simulink model "Car"  (R2024b)
settings: Solver=ode15s  StartTime=0.0  StopTime=PROFILE_LENGTH  MaxStep=300  RelTol=1e-7
values from neighbouring files (symbols this model uses):
  ACCEL_TOLERANCE = 1    [Setup.m]
  AIR_DENSITY = 1.2    [Setup.m]
  C_ROLLING_RESISTANCE = .0025    (= 0.0025)    [Setup.m]
  CONTROL_MODE = 1    [Setup.m]
  CURRENT_DATA_ECO = ECO_DATA(:, 1)    [Setup.m]
  CURRENT_DATA_POWER = POWER_DATA(:, 1)    [Setup.m]
  D_POWER = 1    [Setup.m]
  D_SPEED = 40    [Setup.m]
  DRAG_COEFFICIENT = 0.25    [Setup.m]
  DRIVER_DISPLAY_DRAW = 2.5    [Setup.m]
  FAN_DRAW = 4.8    [Setup.m]
  FORECASTED_IRRADIANCE = -5*((SOLAR_TIME_BREAKPOINTS-START_TIME).*(SOLAR_TIME_BREAKPOINTS-END_TIME) / (PROFILE_LENGTH/2)^2)    [Setup.m]
  FRONTAL_AREA = 1    [Setup.m]
  FULL_PACK_KWH = HV_PACK_VOLTAGE * HV_PACK_CAPACITY * UNIT_TO_KILO    (= 7.68)    [Setup.m]
  GRAVITY = 9.81    [Setup.m]
  HEADLIGHT_DRAW = 2    [Setup.m]
  HV_PACK_VOLTAGE = 96    [Setup.m]
  I_POWER = 1    [Setup.m]
  I_SPEED = 3    [Setup.m]
  INT_DISTANCES = COURSE_DATA(:, 8) / UNIT_TO_KILO    [Setup.m]
  INT_GRADE_ANGLE = rad2deg(atan(COURSE_DATA(:, 7)/100))    [Setup.m]
  MAX_CURRENT_ECO = max(CURRENT_DATA_ECO)    [Setup.m]
  MAX_CURRENTS_ECO = flip(CURRENT_DATA_ECO)    [Setup.m]
  MAX_CURRENTS_POWER = flip(CURRENT_DATA_POWER)    [Setup.m]
  P_POWER = 10    [Setup.m]
  P_SPEED = 25    [Setup.m]
  REGEN_ON = 0    [Setup.m]
  RPM_BREAKPOINTS_ECO = flip(RPM_DATA_ECO)    [Setup.m]
  RPM_BREAKPOINTS_POWER = flip(RPM_DATA_POWER)    [Setup.m]
  RPM_DATA_ECO = ECO_DATA(:, 3)    [Setup.m]
  RPM_DATA_POWER = POWER_DATA(:, 3)    [Setup.m]
  SECONDS_PER_HOUR = 3600    [Setup.m]
  SOLAR_TIME_BREAKPOINTS = START_TIME:900:END_TIME    [Setup.m]
  SPEED_TO_RPM = 60 / (WHEEL_DIAMETER_METERS * pi)    (= 34.1778689532)    [Setup.m]
  START_TIME = CURRENT_TIME    [Setup.m]
  STARTING_KWH = FULL_PACK_KWH * (1 - 0)    (= 7.68)    [Setup.m]
  TARGET_POWER = 700    [Setup.m]
  TARGET_SPEED = 12    [Setup.m]
  TORQUES_DATA_ECO = ECO_DATA(:, 2)    [Setup.m]
  TORQUES_DATA_POWER = POWER_DATA(:, 2) * 2.5    [Setup.m]
  TOTAL_MASS = CAR_MASS + DRIVER_MASS    (= 282.996279643)    [Setup.m]
  UNIT_TO_KILO = 1 / 1000    (= 0.001)    [Setup.m]
  WHEEL_RADIUS = WHEEL_DIAMETER_METERS / 2    (= 0.2794)    [Setup.m]
undefined symbols (not defined in the file or in its folder): density, density_elevation, distance, elevation, INT_CURRENTS, INT_TORQUES_ECO, MAX_TORQUE
libraries: slpidlib x4, simulink x1
(part 2 of 2)

== system Car/Control/Filter if below min SOC/Control Mode/Speed Control ==
  Speed : Inport
  Target Speed : Inport  Port=2
  Action Port : ActionPort  ActionPortLabel=if(u1 == 0)
  PID Controller1 : slpidlib/PID Controller  Controller=PID  Form=Parallel  TimeDomain=Continuous-time  UseExternalTs=off  SampleTime=-1  IntegratorMethod=Forward Euler  FilterMethod=Forward Euler  ControllerParametersSource=internal  P=P_SPEED  I=I_SPEED  UseKiTs=off  D=D_SPEED  UseExternalDerivativeSource=off  N=100  UseFilter=on  TunerSelectOption=Transfer Function Based (PID Tuner App)  InitialConditionSource=internal  InitialConditionForIntegrator=0  InitialConditionForFilter=0  DifferentiatorICPrevScaledInput=0  ExternalReset=none  TrackingMode=off  Kt=1  LimitOutput=off  SatLimitsSource=internal  UpperSaturationLimit=inf  LowerSaturationLimit=-inf  LinearizeAsGain=on  AntiWindupMode=none  Kb=1  LimitIntegrator=off  UpperIntegratorSaturationLimit=inf  LowerIntegratorSaturationLimit=-inf  POutMin=[]  POutMax=[]  IOutMin=[]  IOutMax=[]  DOutMin=[]  DOutMax=[]  NOutMin=[]  NOutMax=[]  SumOutMin=[]  SumOutMax=[]  SaturationOutMin=[]  SaturationOutMax=[]  PParamMin=[]  PParamMax=[]  IParamMin=[]  IParamMax=[]  DParamMin=[]  DParamMax=[]  NParamMin=[]  NParamMax=[]  KbParamMin=[]  KbParamMax=[]  KtParamMin=[]  KtParamMax=[]  KbOutMin=[]  KbOutMax=[]  KtOutMin=[]  KtOutMax=[]  IntegratorOutMin=[]  IntegratorOutMax=[]  FilterOutMin=[]  FilterOutMax=[]  SumI1OutMin=[]  SumI1OutMax=[]  SumI2OutMin=[]  SumI2OutMax=[]  SumI3OutMin=[]  SumI3OutMax=[]  SumI4OutMin=[]  SumI4OutMax=[]  SumDOutMin=[]  SumDOutMax=[]  DifferentiatorOutMin=[]  DifferentiatorOutMax=[]  FilterDiffOutCoefMin=[]  FilterDiffOutCoefMax=[]  ReciprocalOutMin=[]  ReciprocalOutMax=[]  SumDenOutMin=[]  SumDenOutMax=[]  SumNumOutMin=[]  SumNumOutMax=[]  DivideOutMin=[]  DivideOutMax=[]  UdiffTsProdOutMin=[]  UdiffTsProdOutMax=[]  NTsProdOutMin=[]  NTsProdOutMax=[]  UintegralTsProdOutMin=[]  UintegralTsProdOutMax=[]  UngainTsProdOutMin=[]  UngainTsProdOutMax=[]  ClampingZeroOutDataTypeStr=Inherit: Inherit via back propagation  ClampingZeroOutMin=[]  ClampingZeroOutMax=[]  FilterDenConstantOutDataTypeStr=Inherit: Inherit via back propagation  FilterDenConstantOutMin=[]  FilterDenConstantOutMax=[]  PCopyOutDataTypeStr=Inherit: Inherit via back propagation  PCopyOutMin=[]  PCopyOutMax=[]  NCopyOutDataTypeStr=Inherit: Inherit via back propagation  NCopyOutMin=[]  NCopyOutMax=[]  IntegratorContinuousStateAttributes=''  IntegratorStateMustResolveToSignalObject=off  IntegratorRTWStateStorageClass=Auto  FilterContinuousStateAttributes=''  FilterStateMustResolveToSignalObject=off  FilterRTWStateStorageClass=Auto  ParallelPVariant=InternalParameters  IdealPVariant=Disabled  IVariant=InternalParameters  DVariant=InternalParameters  IntegratorVariant=Continuous  SatVariant=Disabled  AWVariant=Passthrough  PCopyVariant=Disabled  TRVariant=Disabled  FdbkBlocksVariant=Forward  IdealPFdbkVariant=Disabled  SatFdbkVariant=Disabled  DerivativeFilterVariant=ContFilter  NVariant=InternalParameters  NCopyVariant=Disabled  FilterICVariant=InternalICsFilter  IntegratorICVariant=InternalICs  ExternalResetVariant=Disabled  TRSumVariant=Passthrough  SumFdbkVariant=Disabled  SumVariant=Sum_PID  TsampFilterVariant=InternalTs  TsampNgainVariant=Passthrough  TsampIntegralVariant=Disabled_SignalSpec  ExternalSaturationOutDataTypeStr=Inherit: Same as second input  DerivativeSourceVariant=ErrorSignal  PreIntVariant=InternalPreInt
  Subtract : Sum  Inputs=-+
  Out1 : Outport
  wires:
  Speed/1 -> Subtract/1
  PID Controller1/1 -> Out1/1  "ControlSpeedSignal"
  Subtract/1 -> PID Controller1/1  "SpeedError"
  Target Speed/1 -> Subtract/2

== system Car/Control/Limit Maximum Current/If Action Subsystem/If Action Subsystem ==
  Action Port : ActionPort
  Constant : Constant  Value=MAX_CURRENT_ECO
  Out1 : Outport
  wires:
  Constant/1 -> Out1/1

== system Car/Control/Limit Maximum Current/If Action Subsystem/If Action Subsystem1 ==
  RPM : Inport
  Action Port : ActionPort
  1-D Lookup Table : Lookup_n-D  NumberOfTableDimensions=1  BreakpointsForDimension1=RPM_DATA_ECO  Table=CURRENT_DATA_ECO  ExtrapMethod=Clip  DiagnosticForOutOfRangeInput=Warning  InternalRulePriority=Speed  RndMeth=Simplest
  MaxCurrentEco : Outport
  wires:
  RPM/1 -> 1-D Lookup Table/1
  1-D Lookup Table/1 -> MaxCurrentEco/1

== system Car/Control/Limit Maximum Current/If Action Subsystem1/If Action Subsystem ==
  Action Port : ActionPort  ActionPortLabel=if(u1 > MAX_RPM_ECO)
  Constant : Constant  Value=MAX_CURRENT_ECO
  Out1 : Outport
  wires:
  Constant/1 -> Out1/1

== system Car/Control/Limit Maximum Current/If Action Subsystem1/If Action Subsystem1 ==
  RPM : Inport
  Action Port : ActionPort  ActionPortLabel=else
  1-D Lookup Table : Lookup_n-D  NumberOfTableDimensions=1  BreakpointsForDimension1=RPM_DATA_POWER  Table=CURRENT_DATA_POWER  ExtrapMethod=Clip  DiagnosticForOutOfRangeInput=Warning  InternalRulePriority=Speed  RndMeth=Simplest
  MaxCurrentEco : Outport
  wires:
  RPM/1 -> 1-D Lookup Table/1
  1-D Lookup Table/1 -> MaxCurrentEco/1

== system Car/Forces/Propulsion (Motor)/Curent Cap/lookup maximum eco mode current ==
  note: Eco Mode
  RPM : Inport
  Action Port : ActionPort  ActionPortLabel=if(u1 ~= 1)
  1-D Lookup Table : Lookup_n-D  NumberOfTableDimensions=1  BreakpointsForDimension1=RPM_BREAKPOINTS_ECO  IndexSearchMethod=Linear search  Table=MAX_CURRENTS_ECO  ExtrapMethod=Clip  InternalRulePriority=Speed  RndMeth=Simplest
  MaxCurrentEco : Outport
  wires:
  RPM/1 -> 1-D Lookup Table/1
  1-D Lookup Table/1 -> MaxCurrentEco/1  "MaxCurrentEco"

== system Car/Forces/Propulsion (Motor)/Curent Cap/lookup maximum power mode current ==
  RPM : Inport
  Action Port : ActionPort  ActionPortLabel=else
  1-D Lookup Table : Lookup_n-D  NumberOfTableDimensions=1  BreakpointsForDimension1=RPM_BREAKPOINTS_POWER  IndexSearchMethod=Linear search  Table=MAX_CURRENTS_POWER  ExtrapMethod=Clip  InternalRulePriority=Speed  RndMeth=Simplest
  MaxCurrentPower : Outport
  wires:
  RPM/1 -> 1-D Lookup Table/1
  1-D Lookup Table/1 -> MaxCurrentPower/1

== system Car/Forces/Propulsion (Motor)/Torque Production/If Action Subsystem ==
  note: Eco Mode
  current : Inport
  Action Port : ActionPort  ActionPortLabel=if(u1 ~= 1)
  1-D Lookup Table : Lookup_n-D  NumberOfTableDimensions=1  BreakpointsForDimension1=CURRENT_DATA_ECO  Table=TORQUES_DATA_ECO  ExtrapMethod=Clip  InternalRulePriority=Speed  RndMeth=Simplest
  torqueEco : Outport
  wires:
  current/1 -> 1-D Lookup Table/1
  1-D Lookup Table/1 -> torqueEco/1

== system Car/Forces/Propulsion (Motor)/Torque Production/If Action Subsystem1 ==
  note: Power Mode
  current : Inport
  Action Port : ActionPort  ActionPortLabel=else
  1-D Lookup Table : Lookup_n-D  NumberOfTableDimensions=1  BreakpointsForDimension1=CURRENT_DATA_POWER  IndexSearchMethod=Linear search  Table=TORQUES_DATA_POWER  ExtrapMethod=Clip  InternalRulePriority=Speed  RndMeth=Simplest
  torqueEco : Outport
  wires:
  current/1 -> 1-D Lookup Table/1
  1-D Lookup Table/1 -> torqueEco/1

== matlab function Car/Course Parameters/MATLAB Function ==
  data: temperature input; density output; pressure input; humidity input; viscosity output
function [density, viscosity] = air(temperature, pressure, humidity)
    [density, viscosity] = airParams(temperature, pressure, humidity);
end
